simulink model "constants"  (R2013a)
settings: Solver=ode45  StartTime=0.0  StopTime=10.0  RelTol=1e-3
StartFcn:
  | % This is the StartFcn callback for a Simulink model
  | 
  | % name of the open model
  | model_name = bdroot();
  | 
  | % get all blocks
  | blks = find_system('adder', 'Type', 'Block');
  | 
  | % add listener to each block
  | disp('Adding callbacks')
  | 
  | for i = 1:length(blks)
  | 	disp(blks{i});
  | 	listener{i} = add_exec_event_listener(blks{i}, 'PostOutputs', @blockCallback);
  | end
  | 
  | disp('Callbacks added')
settings Model: Creator=Sunil  LastModifiedBy=Sunil

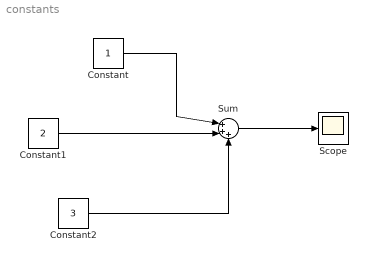
== system constants ==
  Constant : Constant
  Constant1 : Constant  Value=2
  Constant2 : Constant  Value=3
  Scope : Scope
  Sum : Sum  Inputs=|+++
  wires:
  Constant/1 -> Sum/1
  Sum/1 -> Scope/1
  Constant1/1 -> Sum/2
  Constant2/1 -> Sum/3
